simulink subsystem "Compute_RelState"  (R2023a)
settings: Solver=VariableStepAuto  StartTime=0.0  StopTime=10.0  RelTol=1e-3
libraries: matrix_library x1
settings Model: Creator=Andy  LastModifiedBy=Andy

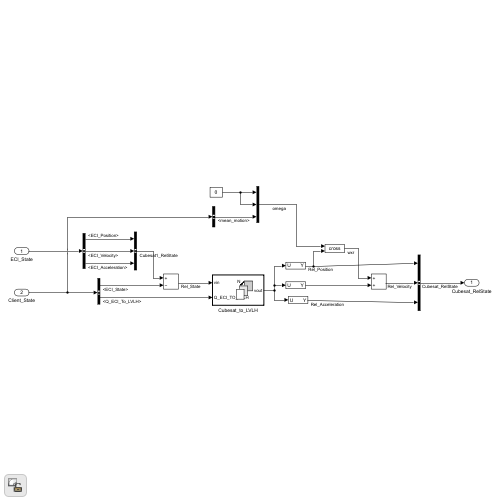
[thumbnail: Simulink's stored preview of the top-level diagram]
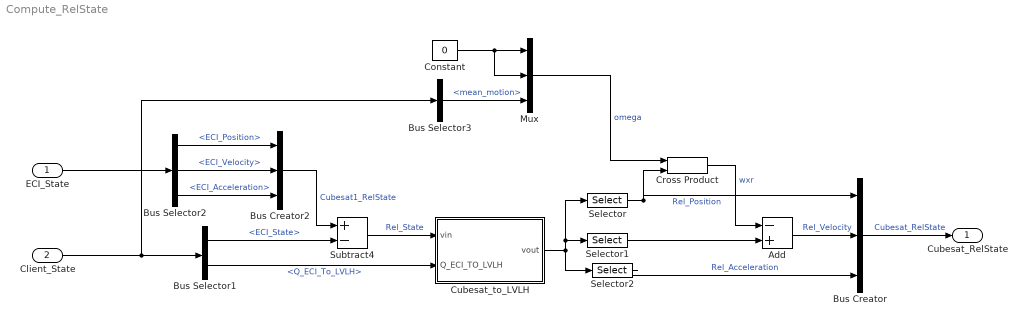
== system Compute_RelState ==
  ECI_State : Inport
  Client_State : Inport  Port=2
  Add : Sum  Inputs=-+
  Bus Creator : BusCreator  Inputs=3
  Bus Creator2 : BusCreator  Inputs=3
  Bus Selector1 : BusSelector  OutputSignals=ECI_State,LVLH_State.Q_ECI_To_LVLH
  Bus Selector2 : BusSelector  OutputSignals=ECI_Position,ECI_Velocity,ECI_Acceleration
  Bus Selector3 : BusSelector  OutputSignals=mean_motion
  Constant : Constant  Value=0
  Cross Product : matrix_library/Cross Product
  Cubesat_to_LVLH : Subsystem  TreatAsAtomicUnit=on
  Mux : Mux  Inputs=3
  Selector : Selector  InputPortWidth=9  IndexOptions=Index vector (dialog)  Indices=[1:3]  OutputSizes=1
  Selector1 : Selector  InputPortWidth=9  IndexOptions=Index vector (dialog)  Indices=[4:6]  OutputSizes=1
  Selector2 : Selector  InputPortWidth=9  IndexOptions=Index vector (dialog)  Indices=[7:9]  OutputSizes=1
  Subtract4 : Sum  Inputs=+-
  Cubesat_RelState : Outport
  wires:
  Bus Selector2/1 -> Bus Creator2/1  "<ECI_Position>"
  Bus Selector2/2 -> Bus Creator2/2  "<ECI_Velocity>"
  Bus Creator2/1 -> Subtract4/1  "Cubesat1_RelState"
  Selector/1 -> Cross Product/2, Bus Creator/1  "Rel_Position"
  Cubesat_to_LVLH/1(vout) -> Selector2/1, Selector1/1, Selector/1
  Bus Selector2/3 -> Bus Creator2/3  "<ECI_Acceleration>"
  Selector2/1 -> Bus Creator/3  "Rel_Acceleration"
  Subtract4/1 -> Cubesat_to_LVLH/1(vin)  "Rel_State"
  ECI_State/1 -> Bus Selector2/1
  Bus Creator/1 -> Cubesat_RelState/1  "Cubesat_RelState"
  Client_State/1 -> Bus Selector1/1, Bus Selector3/1
  Bus Selector1/1 -> Subtract4/2  "<ECI_State>"
  Bus Selector3/1 -> Mux/3  "<mean_motion>"
  Constant/1 -> Mux/1, Mux/2
  Mux/1 -> Cross Product/1  "omega"
  Add/1 -> Bus Creator/2  "Rel_Velocity"
  Cross Product/1 -> Add/1  "wxr"
  Selector1/1 -> Add/2
  Bus Selector1/2 -> Cubesat_to_LVLH/2(Q_ECI_TO_LVLH)  "<Q_ECI_To_LVLH>"

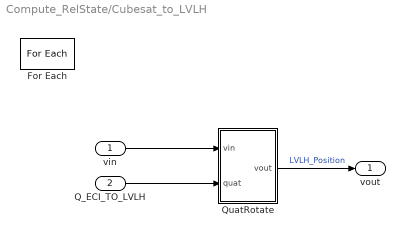
== system Compute_RelState/Cubesat_to_LVLH ==
  vin : Inport  Partition=on  PartitionDimension=1  PartitionWidth=3  PartitionOffset=0
  Q_ECI_TO_LVLH : Inport  Port=2
  For Each : ForEach  DisableCoverage=on
  QuatRotate : MATLAB Function  TreatAsAtomicUnit=on
  vout : Outport  ConcatenationDimension=1
  wires:
  QuatRotate/1(vout) -> vout/1  "LVLH_Position"
  vin/1 -> QuatRotate/1(vin)
  Q_ECI_TO_LVLH/1 -> QuatRotate/2(quat)

== matlab function Compute_RelState/Cubesat_to_LVLH/QuatRotate ==
  data: vin input; vout output; quat input
function vout = fcn(vin,quat)

vout = quatrotate(vin,quat);
